simulink model "flbk"  (R2023b)
settings: Solver=VariableStepAuto  StartTime=0.0  StopTime=10.0  RelTol=1e-3
undefined symbols (not defined in the file): c, l
libraries: spsSeriesRLCBranchLib x3, spsCurrentMeasurementLib x2, spsDCVoltageSourceLib x1, spsDiodeLib x1, spsIGBTDiodeLib x1, spsLinearTransformerLib x1, spsVoltageMeasurementLib x1, simulink x1, spspowerguiLib x1
settings Model: Creator=91798  LastModifiedBy=91798

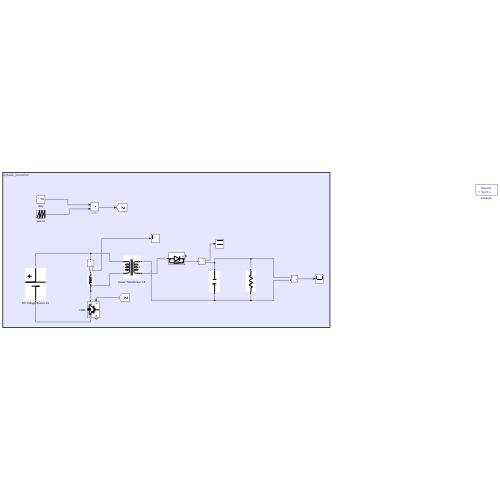
[thumbnail: Simulink's stored preview of the top-level diagram]
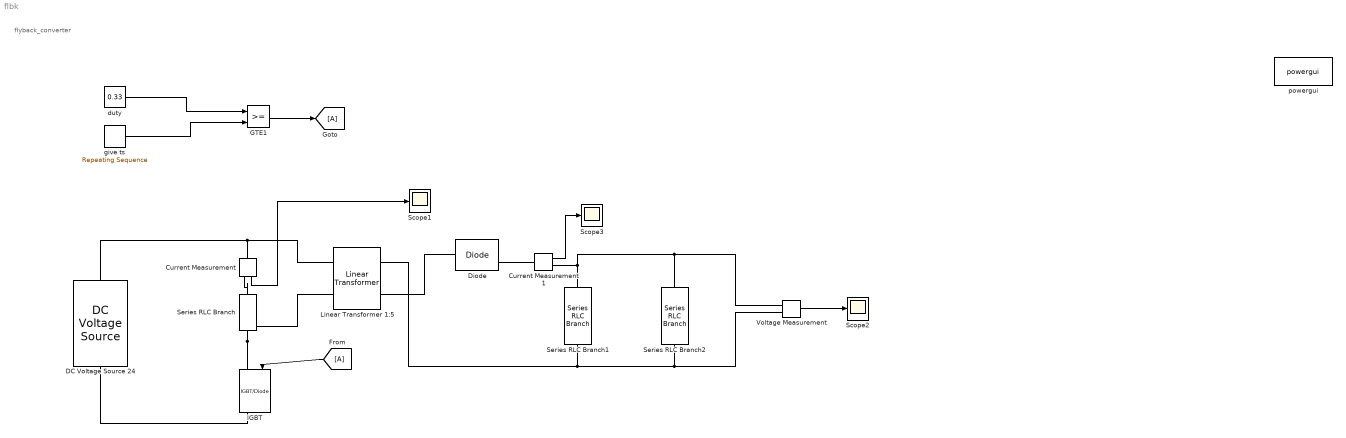
== system flbk ==
  note: flyback_converter
  Current Measurement : spsCurrentMeasurementLib/Current Measurement  PhasorSimulation=off  OutputType=Complex  PSBequivalent=0
  Current Measurement1 : spsCurrentMeasurementLib/Current Measurement  PhasorSimulation=off  OutputType=Complex  PSBequivalent=0
  DC Voltage Source 24 : spsDCVoltageSourceLib/DC Voltage Source  Amplitude=24  Measurements=Voltage
  Diode : spsDiodeLib/Diode  Ron=0.0001  Lon=0  Vf=0.8  IC=0  UseSnubber=0  Rs=500  Cs=250e-9  Measurements=on
  From : From
  GTE1 : RelationalOperator  OutDataTypeStr=boolean  RndMeth=Simplest  InputSameDT=off
  Goto : Goto
  IGBT : spsIGBTDiodeLib/IGBT//Diode  Ron=1e-6  Rs=1e5  Cs=inf  Measurements=on
  Linear Transformer 1:5 : spsLinearTransformerLib/Linear Transformer  UNITS=SI  NominalPower=[ 250e6 20e3 ]  winding1=[24 0 0]  winding2=[120 0 0]  ThreeWindings=off  winding3=[3.15e+05 0.7938 0.084225]  RmLm=[1e6 inf]  Measurements=None  DataType=on
  Scope1 : Scope
  Scope2 : Scope
  Scope3 : Scope
  Series RLC Branch : spsSeriesRLCBranchLib/Series RLC Branch  LConnTagsString=__new0  RConnTagsString=__new0  BranchType=L  Resistance=1  Inductance=l  SetiL0=off  InitialCurrent=0  Capacitance=1e-6  Setx0=off  InitialVoltage=0  Measurements=None
  Series RLC Branch1 : spsSeriesRLCBranchLib/Series RLC Branch  LConnTagsString=__new0  RConnTagsString=__new0  BranchType=C  Resistance=1  Inductance=1e-3  SetiL0=off  InitialCurrent=0  Capacitance=c  Setx0=off  InitialVoltage=0  Measurements=None
  Series RLC Branch2 : spsSeriesRLCBranchLib/Series RLC Branch  LConnTagsString=__new0  RConnTagsString=__new0  BranchType=R  Resistance=5  Inductance=1e-3  SetiL0=off  InitialCurrent=0  Capacitance=1e-6  Setx0=off  InitialVoltage=0  Measurements=None
  Voltage Measurement : spsVoltageMeasurementLib/Voltage Measurement  PhasorSimulation=off  OutputType=Complex  PSBequivalent=0
  duty : Constant  Value=0.33
  give ts : simulink/Sources/Repeating Sequence  rep_seq_t=[0 5e-5]  rep_seq_y=[0 1]
  powergui : spspowerguiLib/powergui  Priority=1  SimulationMode=Discrete  SampleTime=5e-7  frequency=60  Iterations=50  frequencyindice=0  Pbase=100e6  ErrMax=1e-4  UnitsV=kV  UnitsW=MW  buscounter=0  FunctionMessages=off  echomessages=off  EnableUseOfTLC=off  CurrentSourceSwitches=off  DisableSnubberDevices=off  DisableRonSwitches=off  DisableVfSwitches=off  DisplayEquations=off  AutomaticDiscreteSolvers=off  SolverType=Tustin/Backward Euler (TBE)  Interpol=off  ExternalGateDelay=off  methode=off  Ts=100  x0status=blocks  SPID=on  SwTol=0  HookPort=off  NonlinearTolerance=1e-4  nMaxIteration=100  ContinueOnMaxIteration=off  RestoreLinks=warning  ResistiveCurrentMeasurement=off  Frange=[0:2:500]  Ylog=off  Xlog=on  ShowGrid=off  save=off  variable=ZData  structure=0  ZoomFFT=off  StartTime=0.0  cycles=1  DisplayStyle=1  fundamental=60  FreqAxis=off  MaxFrequency=1000  frequencyindicesteady=1  RmsSteady=1  display=off
  wires:
  Current Measurement/1 -> Scope1/1
  Voltage Measurement/1 -> Scope2/1
  give ts/1 -> GTE1/2
  duty/1 -> GTE1/1
  GTE1/1 -> Goto/1
  From/1 -> IGBT/1
  Current Measurement1/1 -> Scope3/1
  connections:
  Series RLC Branch1/RConn1 -- Series RLC Branch2/RConn1 -- Voltage Measurement/LConn2 -- Linear Transformer 1:5/RConn1
  Series RLC Branch2/LConn1 -- Voltage Measurement/LConn1 -- Current Measurement1/RConn1 -- Series RLC Branch1/LConn1
  Series RLC Branch/RConn1 -- Linear Transformer 1:5/LConn2 -- IGBT/LConn1
  Current Measurement/LConn1 -- Linear Transformer 1:5/LConn1 -- DC Voltage Source 24/RConn1
  DC Voltage Source 24/LConn1 -- IGBT/RConn1
  Linear Transformer 1:5/RConn2 -- Diode/LConn1
  Series RLC Branch/LConn1 -- Current Measurement/RConn1
  Current Measurement1/LConn1 -- Diode/RConn1
